simulink model "Queue_en_Model"  (R2024b)
settings: Solver=VariableStepAuto  StartTime=0.0  StopTime=10.0  RelTol=1e-3
libraries: NSA_DEVS_SINKS x5, NSA_DEVS_LOGISTICS x3, NSA_DEVS_SOURCES x2
settings Model: Creator=david  LastModifiedBy=peter
settings RTWCC: GPUComputeCapability=3.5

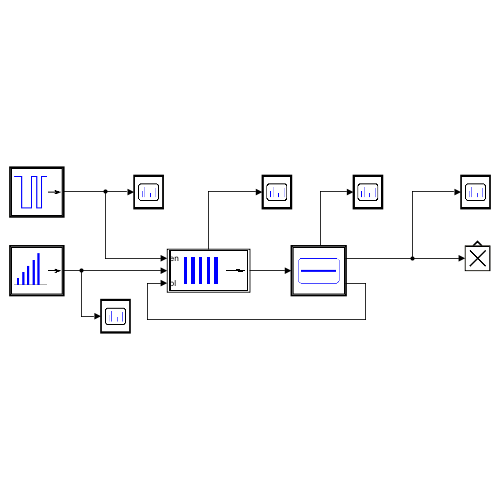
[thumbnail: Simulink's stored preview of the top-level diagram]
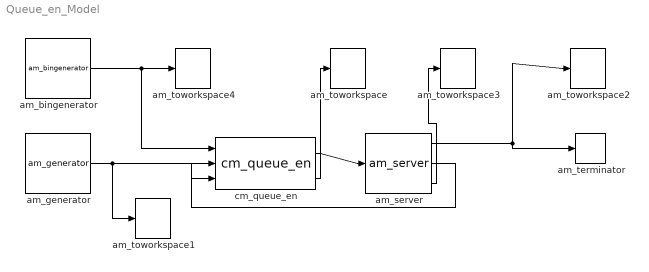
== system Queue_en_Model ==
  am_bingenerator : NSA_DEVS_SOURCES/am_bingenerator  z0=true  tVec=[20.0, 70.0, 110, 120]  tau=[0,1]  debug=0
      settings: SourceProductName=Sources
  am_generator : NSA_DEVS_SOURCES/am_generator  tG=3.0  n0=1  nG=50  tD=[0,2]  debug=0
      settings: SourceProductName=Sources
  am_server : NSA_DEVS_LOGISTICS/am_server  tS=1.5  tsField="\"\""  tau=[0,1]  debug=0
      settings: SourceProductName=Logistics
  am_terminator : NSA_DEVS_LOGISTICS/am_terminator  tau=[0,1]  debug=0
      settings: SourceProductName=Logistics
  am_toworkspace : NSA_DEVS_SINKS/am_toworkspace  varname="\"bufferNQ\""  t0=0  format="\"vector\""  tau=[0,5]  debug=0
      settings: SourceProductName=Sinks
  am_toworkspace1 : NSA_DEVS_SINKS/am_toworkspace  varname="\"genOut\""  t0=0  format="\"vector\""  tau=[0,5]  debug=0
      settings: SourceProductName=Sinks
  am_toworkspace2 : NSA_DEVS_SINKS/am_toworkspace  varname="\"srvOut\""  t0=0  format="\"vector\""  tau=[0,5]  debug=0
      settings: SourceProductName=Sinks
  am_toworkspace3 : NSA_DEVS_SINKS/am_toworkspace  varname="\"srvnOut\""  t0=0  format="\"vector\""  tau=[0,5]  debug=0
      settings: SourceProductName=Sinks
  am_toworkspace4 : NSA_DEVS_SINKS/am_toworkspace  varname="\"bingenOut\""  t0=0  format="\"vector\""  tau=[0,5]  debug=0
      settings: SourceProductName=Sinks
  cm_queue_en : NSA_DEVS_LOGISTICS/cm_queue_en  tau=[0,1]  debug=0
      link override am_queue: tD=tau.*3
      settings: SourceProductName=Logistics
  wires:
  am_generator/1 -> am_toworkspace1/1, cm_queue_en/2
  cm_queue_en/1 -> am_server/1
  am_server/2 -> cm_queue_en/3
  am_bingenerator/1 -> am_toworkspace4/1, cm_queue_en/1
  am_server/1 -> am_terminator/1, am_toworkspace2/1
  cm_queue_en/2 -> am_toworkspace/1
  am_server/3 -> am_toworkspace3/1
